simulink library "fdclib6"  (Simulink 2.09)
values from neighbouring files (symbols this model uses):
  GM1 = [cbar b    S    Ix   Iy   Iz   Jxy  Jxz  Jyz  m]    [modbuild.m]
undefined symbols (not defined in the file or in its folder): xinco

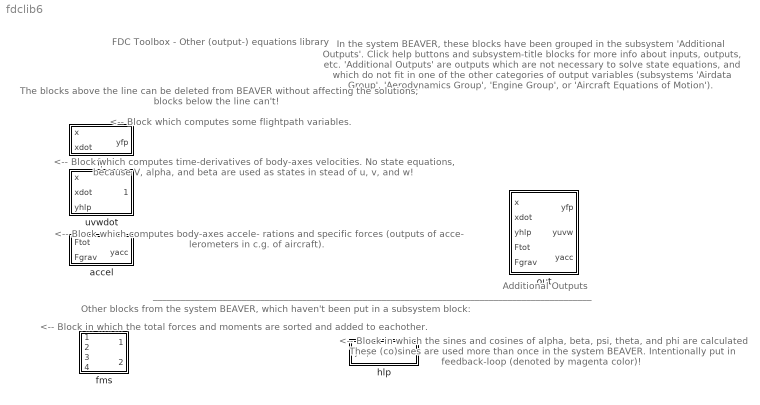
== system fdclib6 ==
  note: In the system BEAVER, these blocks have been grouped
      | in the subsystem 'Additional Outputs'. Click help buttons
      | and subsystem-title blocks for more info about inputs,
      | outputs, etc. 'Additional Outputs' are outputs which are
      | not necessary to solve state equations, and which do
      | not fit in one of the other categories of output variables
      | (subsystems 'Airdata Group', 'Aerodynamics Group',
      | 'Engine Group', or 'Aircraft Equations of Motion').
  note: Additional Outputs
  note: FDC Toolbox - Other (output-) equations library
  note: <-- Block which computes body-axes accele-
      |    rations and specific forces (outputs of acce-
      | lerometers in c.g. of aircraft).
  note: <-- Block which computes time-derivatives
      | of body-axes velocities. No state equations,
      | because V, alpha, and beta are used as
      | states in stead of u, v, and w!
  note: ______________________________________________________________________________________________
  note: The blocks above the line can be deleted from BEAVER
      | without affecting the solutions; blocks below the line can't!
  note: Other blocks from the system BEAVER, which haven't been put in a subsystem block:
  note: <-- Block in which the total forces and
      | moments are sorted and added to
      | eachother.
  note: <-- Block in which the sines and cosines of
      | alpha, beta, psi, theta, and phi are calculated
      | These (co)sines are used more than once in
      | the system BEAVER. Intentionally put in
      | feedback-loop (denoted by magenta color)!
  note: <-- Block which computes some
      | flightpath variables.
  accel : Subsystem  mask(accel){m=GM1(10)}
      mask prompts: m "Mass of the aircraft [kg]:"
      mask help:
      | Body axes accelerations and
      | specific forces.
      mask Help: eval('fdchelp accel')
      mask Display: disp('Accel')
  fms : Subsystem
      mask Type: FMsort
      mask Description: Forces and Moments sorting block
      mask Help: eval('fdchelp fmsort')
      mask Display: disp('FMsort')
  fp : Subsystem  mask(Flpath){alpha0=xinco(2)}
      mask prompts: alpha0 "Initial value of angle of attack, alpha0:"
      mask help: Flightpath related parameters.
      mask Help: eval('fdchelp flpath')
      mask Display: disp('flpath')
  hlp : Subsystem  Orientation=left
      mask Type: Hlpfcn
      mask Description: Help sines and cosines
      mask Help: eval('fdchelp hlpfcn')
      mask Display: disp('hlpfcn')
  out : Subsystem
  uvwdot : Subsystem
      mask Type: uvwdot
      mask Description: Calculation of du/dt, dv/dt, and dw/dt.
      mask Help: eval('fdchelp uvwdot')
      mask Display: disp('uvwdot')

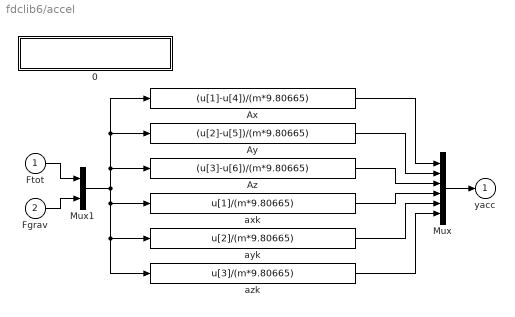
== system fdclib6/accel ==
  Ftot : Inport  Port=1  PortWidth=-1  SampleTime=-1
  Fgrav : Inport  Port=2  PortWidth=-1  SampleTime=-1
  0 : Subsystem
      settings: OpenFcn=fdchelp accel
      mask Display: disp('ACCEL\nM.O. Rauw, October 1997')
  Ax : Fcn  Expr=(u[1]-u[4])/(m*9.80665)
  Ay : Fcn  Expr=(u[2]-u[5])/(m*9.80665)
  Az : Fcn  Expr=(u[3]-u[6])/(m*9.80665)
  Mux : Mux  Inputs=6
  Mux1 : Mux  Inputs=[3 3]
  axk : Fcn  Expr=u[1]/(m*9.80665)
  ayk : Fcn  Expr=u[2]/(m*9.80665)
  azk : Fcn  Expr=u[3]/(m*9.80665)
  yacc : Outport  Port=1  InitialOutput=0
  wires:
  Ftot/1 -> Mux1/1
  Fgrav/1 -> Mux1/2
  Mux/1 -> yacc/1
  azk/1 -> Mux/6
  Az/1 -> Mux/3
  Ay/1 -> Mux/2
  Ax/1 -> Mux/1
  Mux1/1 -> Az/1, Ax/1, Ay/1, axk/1, azk/1, ayk/1
  axk/1 -> Mux/4
  ayk/1 -> Mux/5

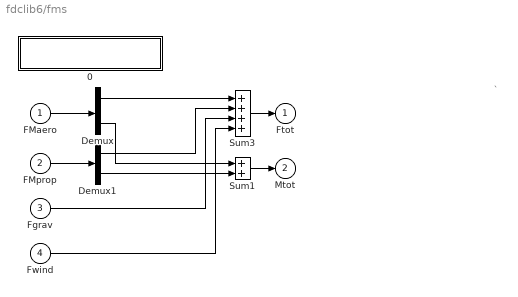
== system fdclib6/fms ==
  note: `
  FMaero : Inport  Port=1  PortWidth=-1  SampleTime=-1
  FMprop : Inport  Port=2  PortWidth=-1  SampleTime=-1
  Fgrav : Inport  Port=3  PortWidth=-1  SampleTime=-1
  Fwind : Inport  Port=4  PortWidth=-1  SampleTime=-1
  0 : Subsystem
      settings: OpenFcn=fdchelp fmsort
      mask Display: disp('FMSORT\nM.O. Rauw, October 1997')
  Demux : Demux  Outputs=[3 3]
  Demux1 : Demux  Outputs=[3 3]
  Sum1 : Sum  Inputs=++
  Sum3 : Sum  Inputs=++++
  Ftot : Outport  Port=1  InitialOutput=0
  Mtot : Outport  Port=2  InitialOutput=0
  wires:
  FMaero/1 -> Demux/1
  FMprop/1 -> Demux1/1
  Demux1/2 -> Sum1/2
  Demux/2 -> Sum1/1
  Fgrav/1 -> Sum3/3
  Demux1/1 -> Sum3/2
  Sum3/1 -> Ftot/1
  Sum1/1 -> Mtot/1
  Demux/1 -> Sum3/1
  Fwind/1 -> Sum3/4

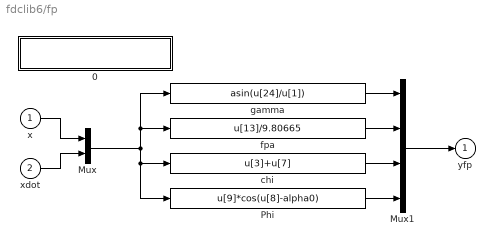
== system fdclib6/fp ==
  x : Inport  Port=1  PortWidth=-1  SampleTime=-1
  xdot : Inport  Port=2  PortWidth=-1  SampleTime=-1
  0 : Subsystem
      settings: OpenFcn=fdchelp flpath
      mask Display: disp('FLPATH\nM.O. Rauw, October 1997')
  Mux : Mux  Inputs=[12 12]
  Mux1 : Mux  Inputs=4
  Phi : Fcn  Expr=u[9]*cos(u[8]-alpha0)
  chi : Fcn  Expr=u[3]+u[7]
  fpa : Fcn  Expr=u[13]/9.80665
  gamma : Fcn  Expr=asin(u[24]/u[1])
  yfp : Outport  Port=1  InitialOutput=0
  wires:
  Mux/1 -> chi/1, Phi/1, fpa/1, gamma/1
  gamma/1 -> Mux1/1
  fpa/1 -> Mux1/2
  chi/1 -> Mux1/3
  Phi/1 -> Mux1/4
  Mux1/1 -> yfp/1
  x/1 -> Mux/1
  xdot/1 -> Mux/2

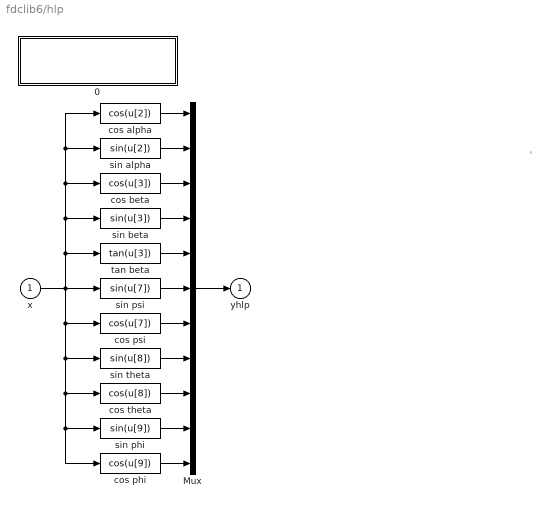
== system fdclib6/hlp ==
  note: '
  x : Inport  Port=1  PortWidth=-1  SampleTime=-1
  0 : Subsystem
      settings: OpenFcn=fdchelp hlpfcn
      mask Display: disp('HELP FUNCTIONS\n(often used sines and cosines)\nM.O. Rauw, October 1997')
  Mux : Mux  Inputs=11
  cos alpha : Fcn  Expr=cos(u[2])
  cos beta : Fcn  Expr=cos(u[3])
  cos phi : Fcn  Expr=cos(u[9])
  cos psi : Fcn  Expr=cos(u[7])
  cos theta : Fcn  Expr=cos(u[8])
  sin alpha : Fcn  Expr=sin(u[2])
  sin beta : Fcn  Expr=sin(u[3])
  sin phi : Fcn  Expr=sin(u[9])
  sin psi : Fcn  Expr=sin(u[7])
  sin theta : Fcn  Expr=sin(u[8])
  tan beta : Fcn  Expr=tan(u[3])
  yhlp : Outport  Port=1  InitialOutput=0
  wires:
  x/1 -> sin psi/1, sin beta/1, cos beta/1, sin alpha/1, cos alpha/1, tan beta/1, sin theta/1, cos theta/1, sin phi/1, cos phi/1, cos psi/1
  cos alpha/1 -> Mux/1
  sin alpha/1 -> Mux/2
  cos beta/1 -> Mux/3
  sin beta/1 -> Mux/4
  tan beta/1 -> Mux/5
  sin psi/1 -> Mux/6
  cos psi/1 -> Mux/7
  sin theta/1 -> Mux/8
  cos theta/1 -> Mux/9
  sin phi/1 -> Mux/10
  Mux/1 -> yhlp/1
  cos phi/1 -> Mux/11

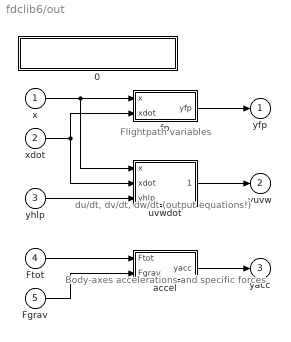
== system fdclib6/out ==
  note: Flightpath
      | variables
  note: du/dt, dv/dt, dw/dt
      | (output equations!)
  note: Body-axes accelerations
      | and specific forces
  x : Inport  Port=1  PortWidth=-1  SampleTime=-1
  xdot : Inport  Port=2  PortWidth=-1  SampleTime=-1
  yhlp : Inport  Port=3  PortWidth=-1  SampleTime=-1
  Ftot : Inport  Port=4  PortWidth=-1  SampleTime=-1
  Fgrav : Inport  Port=5  PortWidth=-1  SampleTime=-1
  0 : Subsystem
      settings: OpenFcn=fdchelp moreouts
      mask Display: disp('Additional outputs (level 3)\nM.O. Rauw')
  accel : Subsystem  mask(accel){m=GM1(10)}
      mask prompts: m "Mass of the aircraft [kg]:"
      mask help:
      | Body axes accelerations and
      | specific forces.
      mask Help: eval('fdchelp accel')
      mask Display: disp('Accel')
  fp : Subsystem  mask(Flpath){alpha0=xinco(2)}
      mask prompts: alpha0 "Initial value of angle of attack, alpha0:"
      mask help: Flightpath related parameters.
      mask Help: eval('fdchelp flpath')
      mask Display: disp('flpath')
  uvwdot : Subsystem
      mask Type: uvwdot
      mask Description: Calculation of du/dt, dv/dt, and dw/dt.
      mask Help: eval('fdchelp uvwdot')
      mask Display: disp('uvwdot')
  yfp : Outport  Port=1  InitialOutput=0
  yuvw : Outport  Port=2  InitialOutput=0
  yacc : Outport  Port=3  InitialOutput=0
  wires:
  fp/1(yfp) -> yfp/1
  uvwdot/1(yuvw =  [udot; vdot; wdot]) -> yuvw/1
  yhlp/1 -> uvwdot/3(yhlp)
  Ftot/1 -> accel/1(Ftot)
  accel/1(yacc) -> yacc/1
  xdot/1 -> fp/2(xdot), uvwdot/2(xdot)
  x/1 -> fp/1(x), uvwdot/1(x)
  Fgrav/1 -> accel/2(Fgrav)

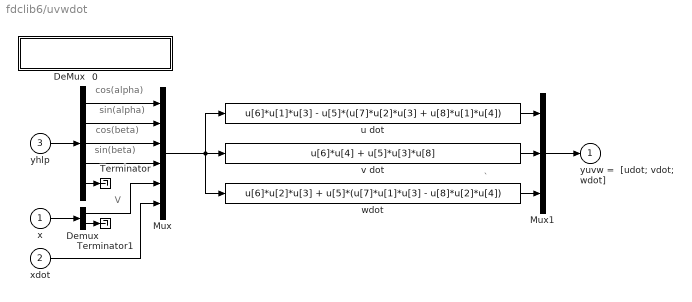
== system fdclib6/uvwdot ==
  note: V
  note: sin(beta)
  note: cos(beta)
  note: sin(alpha)
  note: cos(alpha)
  note: `
  x : Inport  Port=1  PortWidth=-1  SampleTime=-1
  xdot : Inport  Port=2  PortWidth=-1  SampleTime=-1
  yhlp : Inport  Port=3  PortWidth=-1  SampleTime=-1
  0 : Subsystem
      settings: OpenFcn=fdchelp uvwdot
      mask Display: disp('UVWDOT\nM.O. Rauw, October 1997')
  DeMux : Demux  Outputs=[1 1 1 1 7]
  Demux : Demux  Outputs=[1 11]
  Mux : Mux  Inputs=[1 1 1 1 1 12]
  Mux1 : Mux  Inputs=3
  Terminator : Terminator
  Terminator1 : Terminator
  u dot : Fcn  Expr=u[6]*u[1]*u[3] - u[5]*(u[7]*u[2]*u[3] + u[8]*u[1]*u[4])
  v dot : Fcn  Expr=u[6]*u[4] + u[5]*u[3]*u[8]
  wdot : Fcn  Expr=u[6]*u[2]*u[3] + u[5]*(u[7]*u[1]*u[3] - u[8]*u[2]*u[4])
  yuvw =  [udot; vdot; wdot] : Outport  Port=1  InitialOutput=0
  wires:
  Demux/1 -> Mux/5
  DeMux/4 -> Mux/4
  DeMux/3 -> Mux/3
  yhlp/1 -> DeMux/1
  Mux1/1 -> yuvw =  [udot; vdot; wdot]/1
  x/1 -> Demux/1
  DeMux/2 -> Mux/2
  DeMux/1 -> Mux/1
  Mux/1 -> u dot/1, wdot/1, v dot/1
  xdot/1 -> Mux/6
  u dot/1 -> Mux1/1
  v dot/1 -> Mux1/2
  wdot/1 -> Mux1/3
  DeMux/5 -> Terminator/1
  Demux/2 -> Terminator1/1

== system fdclib6/accel/0 ==

== system fdclib6/fms/0 ==

== system fdclib6/fp/0 ==

== system fdclib6/hlp/0 ==

== system fdclib6/out/0 ==

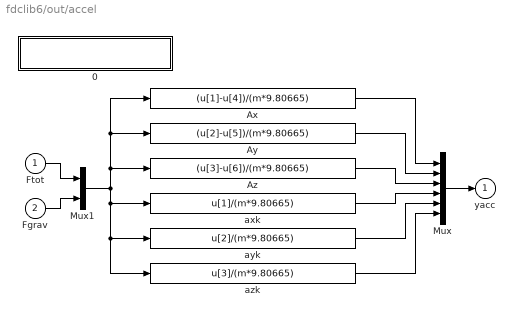
== system fdclib6/out/accel ==
  Ftot : Inport  Port=1  PortWidth=-1  SampleTime=-1
  Fgrav : Inport  Port=2  PortWidth=-1  SampleTime=-1
  0 : Subsystem
      settings: OpenFcn=fdchelp accel
      mask Display: disp('ACCEL\nM.O. Rauw, October 1997')
  Ax : Fcn  Expr=(u[1]-u[4])/(m*9.80665)
  Ay : Fcn  Expr=(u[2]-u[5])/(m*9.80665)
  Az : Fcn  Expr=(u[3]-u[6])/(m*9.80665)
  Mux : Mux  Inputs=6
  Mux1 : Mux  Inputs=[3 3]
  axk : Fcn  Expr=u[1]/(m*9.80665)
  ayk : Fcn  Expr=u[2]/(m*9.80665)
  azk : Fcn  Expr=u[3]/(m*9.80665)
  yacc : Outport  Port=1  InitialOutput=0
  wires:
  Ftot/1 -> Mux1/1
  Fgrav/1 -> Mux1/2
  Mux/1 -> yacc/1
  azk/1 -> Mux/6
  Az/1 -> Mux/3
  Ay/1 -> Mux/2
  Ax/1 -> Mux/1
  Mux1/1 -> Az/1, Ax/1, Ay/1, axk/1, azk/1, ayk/1
  axk/1 -> Mux/4
  ayk/1 -> Mux/5

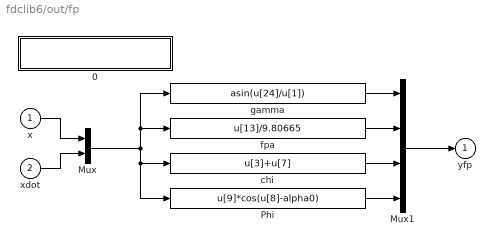
== system fdclib6/out/fp ==
  x : Inport  Port=1  PortWidth=-1  SampleTime=-1
  xdot : Inport  Port=2  PortWidth=-1  SampleTime=-1
  0 : Subsystem
      settings: OpenFcn=fdchelp flpath
      mask Display: disp('FLPATH\nM.O. Rauw, October 1997')
  Mux : Mux  Inputs=[12 12]
  Mux1 : Mux  Inputs=4
  Phi : Fcn  Expr=u[9]*cos(u[8]-alpha0)
  chi : Fcn  Expr=u[3]+u[7]
  fpa : Fcn  Expr=u[13]/9.80665
  gamma : Fcn  Expr=asin(u[24]/u[1])
  yfp : Outport  Port=1  InitialOutput=0
  wires:
  Mux/1 -> chi/1, Phi/1, fpa/1, gamma/1
  gamma/1 -> Mux1/1
  fpa/1 -> Mux1/2
  chi/1 -> Mux1/3
  Phi/1 -> Mux1/4
  Mux1/1 -> yfp/1
  x/1 -> Mux/1
  xdot/1 -> Mux/2

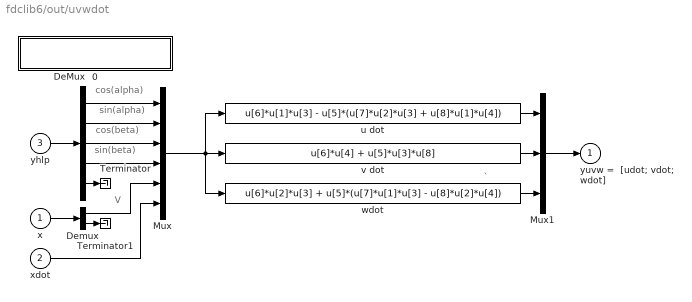
== system fdclib6/out/uvwdot ==
  note: V
  note: sin(beta)
  note: cos(beta)
  note: sin(alpha)
  note: cos(alpha)
  note: `
  x : Inport  Port=1  PortWidth=-1  SampleTime=-1
  xdot : Inport  Port=2  PortWidth=-1  SampleTime=-1
  yhlp : Inport  Port=3  PortWidth=-1  SampleTime=-1
  0 : Subsystem
      settings: OpenFcn=fdchelp uvwdot
      mask Display: disp('UVWDOT\nM.O. Rauw, October 1997')
  DeMux : Demux  Outputs=[1 1 1 1 7]
  Demux : Demux  Outputs=[1 11]
  Mux : Mux  Inputs=[1 1 1 1 1 12]
  Mux1 : Mux  Inputs=3
  Terminator : Terminator
  Terminator1 : Terminator
  u dot : Fcn  Expr=u[6]*u[1]*u[3] - u[5]*(u[7]*u[2]*u[3] + u[8]*u[1]*u[4])
  v dot : Fcn  Expr=u[6]*u[4] + u[5]*u[3]*u[8]
  wdot : Fcn  Expr=u[6]*u[2]*u[3] + u[5]*(u[7]*u[1]*u[3] - u[8]*u[2]*u[4])
  yuvw =  [udot; vdot; wdot] : Outport  Port=1  InitialOutput=0
  wires:
  Demux/1 -> Mux/5
  DeMux/4 -> Mux/4
  DeMux/3 -> Mux/3
  yhlp/1 -> DeMux/1
  Mux1/1 -> yuvw =  [udot; vdot; wdot]/1
  x/1 -> Demux/1
  DeMux/2 -> Mux/2
  DeMux/1 -> Mux/1
  Mux/1 -> u dot/1, wdot/1, v dot/1
  xdot/1 -> Mux/6
  u dot/1 -> Mux1/1
  v dot/1 -> Mux1/2
  wdot/1 -> Mux1/3
  DeMux/5 -> Terminator/1
  Demux/2 -> Terminator1/1

== system fdclib6/uvwdot/0 ==

== system fdclib6/out/accel/0 ==

== system fdclib6/out/fp/0 ==

== system fdclib6/out/uvwdot/0 ==
